simulink model "green_joint_current_loop_twin_model"  (R2023b)
settings: Solver=FixedStepDiscrete  StartTime=0.0  StopTime=GJDT_StopTime  FixedStep=GJDT_TsPlant  RelTol=1e-3
values from neighbouring files (symbols this model uses):
  GJDT_IdRef_A = single(0.0)    [setup_green_joint_current_loop_twin.m]
  GJDT_IqAfter_A = single(0.3)    [run_green_joint_average_motor_twin_smoke_test.m]    (also in run_green_joint_current_loop_saturation_exit_test.m = single(1.5); setup_green_joint_current_loop_twin.m = single(1.5))
  GJDT_IqBefore_A = single(4.0)    [run_green_joint_current_loop_saturation_exit_test.m]    (also in setup_green_joint_current_loop_twin.m = single(0.0))
  GJDT_IqStepTime_s = 0.008    [run_green_joint_current_loop_saturation_exit_test.m]    (also in setup_green_joint_current_loop_twin.m = 0.001)
  GJDT_Ld_H = GJDT_ModuleConfig.phase_inductance_h    [setup_green_joint_current_loop_twin.m]
  GJDT_Lq_H = GJDT_ModuleConfig.phase_inductance_h    [setup_green_joint_current_loop_twin.m]
  GJDT_Rs_Ohm = GJDT_ModuleConfig.phase_resistance_ohm    [setup_green_joint_current_loop_twin.m]
  GJDT_Ts = 50e-6    (= 5e-05)    [setup_green_joint_current_loop_twin.m]
  GJDT_TsPlant = 5e-6    (= 5e-06)    [setup_green_joint_current_loop_twin.m]
  GJDT_Vbus_V = single(12.0)    [setup_green_joint_current_loop_twin.m]
settings Model: DataDictionary=green_joint_current_loop_interface.sldd  Creator=user  LastModifiedBy=user
settings DebuggingCC: ParameterPrecisionLossMsg=none

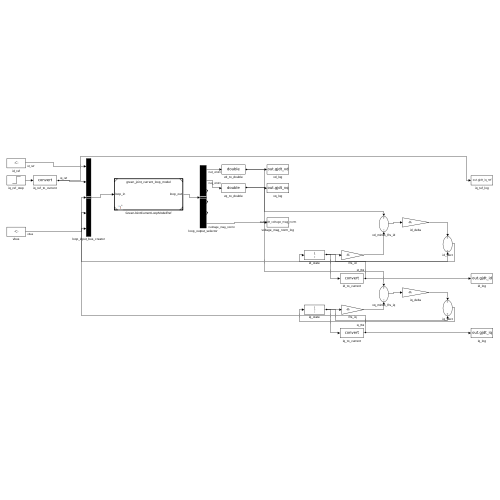
[thumbnail: Simulink's stored preview of the top-level diagram]
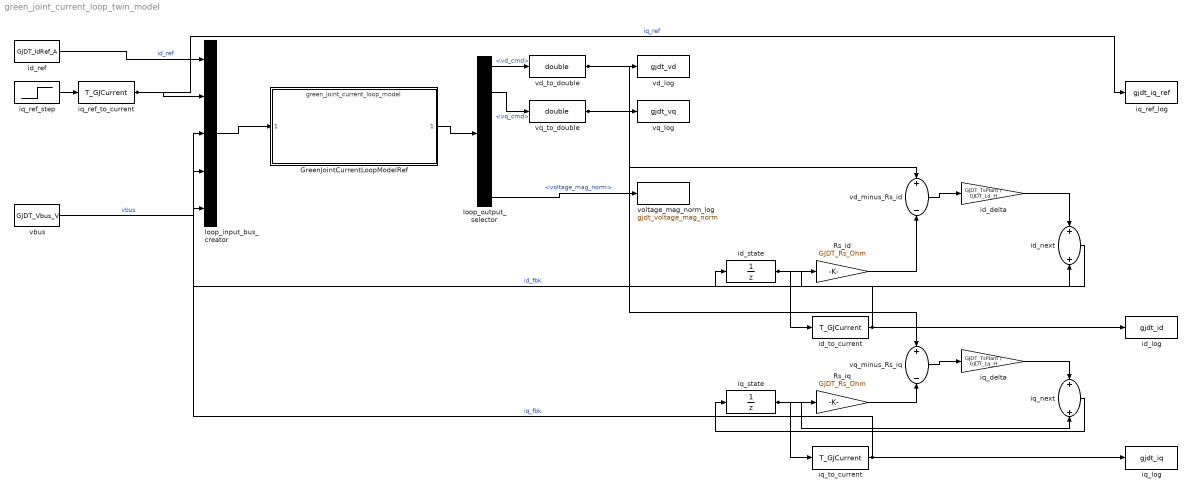
== system green_joint_current_loop_twin_model ==
  GreenJointCurrentLoopModelRef : ModelReference  ModelNameDialog=green_joint_current_loop_model  SimulationMode=Normal  ModelReferenceVersion=1.1
  Rs_id : Gain  Gain=GJDT_Rs_Ohm
  Rs_iq : Gain  Gain=GJDT_Rs_Ohm
  id_delta : Gain  Gain=GJDT_TsPlant / GJDT_Ld_H
  id_log : ToWorkspace  VariableName=gjdt_id  SaveFormat=Structure With Time  SampleTime=-1
  id_next : Sum
  id_ref : Constant  Value=GJDT_IdRef_A  OutDataTypeStr=T_GJCurrent  SampleTime=GJDT_Ts
  id_state : UnitDelay  SampleTime=GJDT_Ts  HasFrameUpgradeWarning=on
  id_to_current : DataTypeConversion  OutDataTypeStr=T_GJCurrent  SaturateOnIntegerOverflow=off  RndMeth=Floor
  iq_delta : Gain  Gain=GJDT_TsPlant / GJDT_Lq_H
  iq_log : ToWorkspace  VariableName=gjdt_iq  SaveFormat=Structure With Time  SampleTime=-1
  iq_next : Sum
  iq_ref_log : ToWorkspace  VariableName=gjdt_iq_ref  SaveFormat=Structure With Time  SampleTime=-1
  iq_ref_step : Step  Time=GJDT_IqStepTime_s  Before=GJDT_IqBefore_A  After=GJDT_IqAfter_A  SampleTime=GJDT_Ts
  iq_ref_to_current : DataTypeConversion  OutDataTypeStr=T_GJCurrent  SaturateOnIntegerOverflow=off  RndMeth=Floor
  iq_state : UnitDelay  SampleTime=GJDT_Ts  HasFrameUpgradeWarning=on
  iq_to_current : DataTypeConversion  OutDataTypeStr=T_GJCurrent  SaturateOnIntegerOverflow=off  RndMeth=Floor
  loop_input_bus_creator : BusCreator  Inputs=5  OutDataTypeStr=Bus: green_joint_current_loop_input_t  NonVirtualBus=on
  loop_output_selector : BusSelector  OutputSignals=vd_cmd,vq_cmd,voltage_mag,vd_norm,vq_norm,voltage_mag_norm
  vbus : Constant  Value=GJDT_Vbus_V  OutDataTypeStr=T_GJVoltage  SampleTime=GJDT_Ts
  vd_log : ToWorkspace  VariableName=gjdt_vd  SaveFormat=Structure With Time  SampleTime=-1
  vd_minus_Rs_id : Sum  Inputs=+-
  vd_to_double : DataTypeConversion  OutDataTypeStr=double  SaturateOnIntegerOverflow=off  RndMeth=Floor
  voltage_mag_norm_log : ToWorkspace  VariableName=gjdt_voltage_mag_norm  SaveFormat=Structure With Time  SampleTime=-1
  vq_log : ToWorkspace  VariableName=gjdt_vq  SaveFormat=Structure With Time  SampleTime=-1
  vq_minus_Rs_iq : Sum  Inputs=+-
  vq_to_double : DataTypeConversion  OutDataTypeStr=double  SaturateOnIntegerOverflow=off  RndMeth=Floor
  wires:
  id_ref/1 -> loop_input_bus_creator/1  "id_ref"
  iq_ref_step/1 -> iq_ref_to_current/1
  iq_ref_to_current/1 -> loop_input_bus_creator/2, iq_ref_log/1  "iq_ref"
  id_to_current/1 -> loop_input_bus_creator/3, id_log/1  "id_fbk"
  iq_to_current/1 -> loop_input_bus_creator/4, iq_log/1  "iq_fbk"
  vbus/1 -> loop_input_bus_creator/5  "vbus"
  loop_input_bus_creator/1 -> GreenJointCurrentLoopModelRef/1
  GreenJointCurrentLoopModelRef/1 -> loop_output_selector/1
  loop_output_selector/1 -> vd_to_double/1  "<vd_cmd>"
  loop_output_selector/2 -> vq_to_double/1  "<vq_cmd>"
  vd_to_double/1 -> vd_minus_Rs_id/1, vd_log/1
  id_state/1 -> Rs_id/1, id_next/2, id_to_current/1
  Rs_id/1 -> vd_minus_Rs_id/2
  vd_minus_Rs_id/1 -> id_delta/1
  id_delta/1 -> id_next/1
  id_next/1 -> id_state/1
  vq_to_double/1 -> vq_minus_Rs_iq/1, vq_log/1
  iq_state/1 -> Rs_iq/1, iq_next/2, iq_to_current/1
  Rs_iq/1 -> vq_minus_Rs_iq/2
  vq_minus_Rs_iq/1 -> iq_delta/1
  iq_delta/1 -> iq_next/1
  iq_next/1 -> iq_state/1
  loop_output_selector/6 -> voltage_mag_norm_log/1  "<voltage_mag_norm>"
